simulink model "uncontrolledRectifier"  (R2021a)
settings: Solver=ode23t  StartTime=0.0  StopTime=.1  FixedStep=.000001  MaxStep=.0001  RelTol=1e-3
undefined symbols (not defined in the file): D1, D11, Delta
libraries: spsVoltageMeasurementLib x49, spsDiodeLib x45, spsCurrentMeasurementLib x21, spsACVoltageSourceLib x20, spsSeriesRLCBranchLib x17, spsMeanLib x3, spsGroundLib x2, spsPowerLib x2, spsThreePhaseTransformerThreeWindingsLib x1, spspowerguiLib x1
settings Model: Creator=User  LastModifiedBy=User

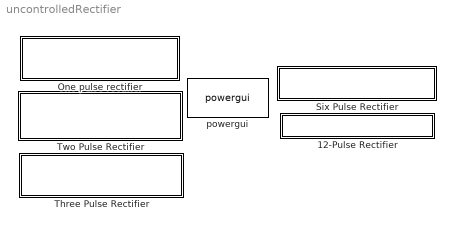
== system uncontrolledRectifier ==
  12-Pulse Rectifier : Subsystem
  One pulse rectifier : Subsystem
  Six Pulse Rectifier : Subsystem
  Three Pulse Rectifier : Subsystem
  Two Pulse Rectifier : Subsystem
  powergui : spspowerguiLib/powergui  Priority=1  SimulationMode=Continuous  SampleTime=50e-6  frequency=60  Iterations=50  frequencyindice=50  Pbase=100e6  ErrMax=1e-4  UnitsV=kV  UnitsW=MW  buscounter=0  FunctionMessages=off  echomessages=off  EnableUseOfTLC=off  CurrentSourceSwitches=off  DisableSnubberDevices=off  DisableRonSwitches=off  DisableVfSwitches=off  DisplayEquations=off  AutomaticDiscreteSolvers=off  SolverType=Tustin/Backward Euler (TBE)  Interpol=off  ExternalGateDelay=off  methode=off  Ts=100  x0status=blocks  SPID=on  SwTol=0  HookPort=off  NonlinearTolerance=1e-4  nMaxIteration=100  ContinueOnMaxIteration=off  RestoreLinks=warning  ResistiveCurrentMeasurement=off  Frange=[0:2:500]  Ylog=off  Xlog=on  ShowGrid=off  save=off  variable=ZData  structure=0  ZoomFFT=off  StartTime=0.0  cycles=1  DisplayStyle=1  fundamental=60  FreqAxis=off  MaxFrequency=1000  frequencyindicesteady=1  RmsSteady=1  display=off

== system uncontrolledRectifier/12-Pulse Rectifier ==
  Subsystem : Subsystem

== system uncontrolledRectifier/One pulse rectifier ==
  Half Wave RL & FWD : Subsystem
  Half Wave RL load : Subsystem
  Half Wave with R : Subsystem
  Half Wave with R//C : Subsystem

== system uncontrolledRectifier/Six Pulse Rectifier ==
  6-pulse with R load : Subsystem
  6-pulse with RL load : Subsystem

== system uncontrolledRectifier/Three Pulse Rectifier ==
  R load : Subsystem

== system uncontrolledRectifier/Two Pulse Rectifier ==
  Full wave with R load : Subsystem
  Full wave with R load And C filter : Subsystem
  Full wave with RL load : Subsystem

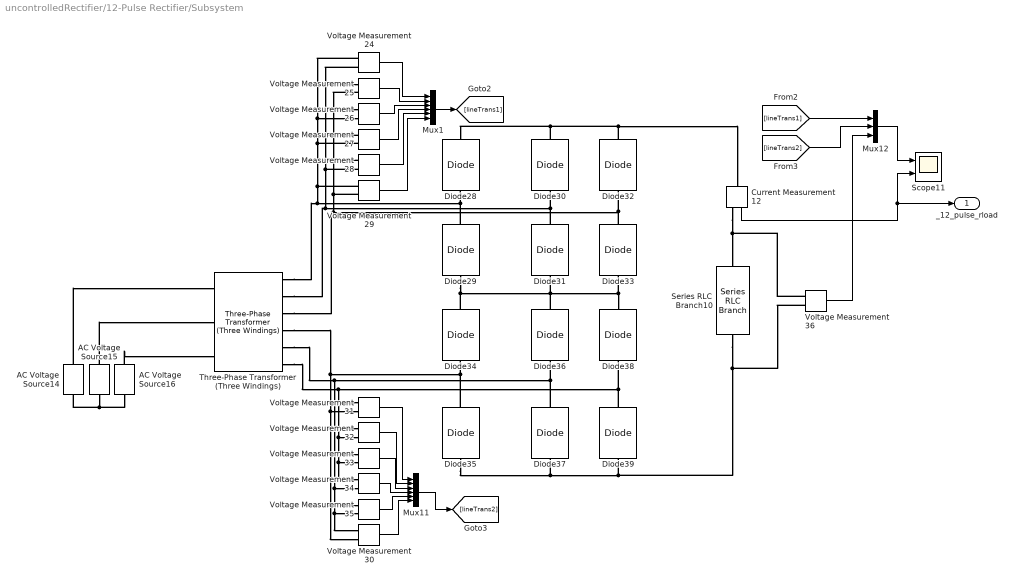
== system uncontrolledRectifier/12-Pulse Rectifier/Subsystem ==
  AC Voltage Source14 : spsACVoltageSourceLib/AC Voltage Source  Amplitude=220*sqrt(2)  Phase=0  Frequency=50  SampleTime=0  Measurements=None  BusType=swing  Pref=10e3  Qref=0  Qmin=-inf  Qmax=+inf
  AC Voltage Source15 : spsACVoltageSourceLib/AC Voltage Source  Amplitude=220*sqrt(2)  Phase=-120  Frequency=50  SampleTime=0  Measurements=None  BusType=swing  Pref=10e3  Qref=0  Qmin=-inf  Qmax=+inf
  AC Voltage Source16 : spsACVoltageSourceLib/AC Voltage Source  Amplitude=220*sqrt(2)  Phase=120  Frequency=50  SampleTime=0  Measurements=None  BusType=swing  Pref=10e3  Qref=0  Qmin=-inf  Qmax=+inf
  Current Measurement12 : spsCurrentMeasurementLib/Current Measurement  PhasorSimulation=off  OutputType=Complex  PSBequivalent=0
  Diode{28..39} (12 alike) : spsDiodeLib/Diode  Ron=0.001  Lon=0  Vf=0.8  IC=0  UseSnubber=0  Rs=500  Cs=250e-9  Measurements=off
  Mux1 : Mux  Inputs=6
  Mux11 : Mux  Inputs=6
  Mux12 : Mux  Inputs=3
  Scope11 : Scope  NumInputPorts=2
  Series RLC Branch10 : spsSeriesRLCBranchLib/Series RLC Branch  LConnTagsString=__new0  RConnTagsString=__new0  BranchType=R  Resistance=10  Inductance=1e-3  SetiL0=off  InitialCurrent=0  Capacitance=1e-6  Setx0=off  InitialVoltage=0  Measurements=None
  Three-Phase Transformer (Three Windings) : spsThreePhaseTransformerThreeWindingsLib/Three-Phase Transformer (Three Windings)  Winding1Connection=Delta (D1)  Winding2Connection=Y  Winding3Connection=Delta (D11)  CoreType=Three single-phase transformers  SetSaturation=off  Hysteresis=off  DataFile='hysteresis'  SetInitialFlux=off  Measurements=None  UNITS=pu  NominalPower=[ 6000 , 50 ]  Winding1=[ 380 , 0.002 , 0.08 ]  Winding2=[ 100 , 0.002 , 0.08 ]  Winding3=[ 100 , 0.002 , 0.08 ]  Rm=500  Lm=500  L0=0.5  Saturation=[ 0,0 ; 0.0024,1.2 ; 1.0,1.52 ]  InitialFluxes=[0.8 -0.8 0.7]  BreakLoop=off  DiscreteSolver=Trapezoidal iterative  DataType=off  TransfoNumber=1
      settings: SourceProductBaseCode=PS
  Voltage Measurement{24..36} (13 alike) : spsVoltageMeasurementLib/Voltage Measurement  PhasorSimulation=off  OutputType=Complex  PSBequivalent=0
  _12_pulse_rload : Outport
  wires:
  Voltage Measurement36/1 -> Mux12/3
  Mux12/1 -> Scope11/1
  Voltage Measurement33/1 -> Mux11/3
  Voltage Measurement24/1 -> Mux1/1
  Voltage Measurement25/1 -> Mux1/2
  Voltage Measurement29/1 -> Mux1/6
  Mux1/1 -> [lineTrans1]
  Voltage Measurement26/1 -> Mux1/3
  Voltage Measurement34/1 -> Mux11/4
  Voltage Measurement30/1 -> Mux11/6
  Voltage Measurement31/1 -> Mux11/1
  Voltage Measurement28/1 -> Mux1/5
  Voltage Measurement35/1 -> Mux11/5
  [lineTrans1] -> Mux12/1
  Mux11/1 -> [lineTrans2]
  Current Measurement12/1 -> _12_pulse_rload/1, Scope11/2
  [lineTrans2] -> Mux12/2
  Voltage Measurement32/1 -> Mux11/2
  Voltage Measurement27/1 -> Mux1/4
  connections:
  Diode37/RConn1 -- Three-Phase Transformer (Three Windings)/RConn5 -- Voltage Measurement33/LConn1 -- Voltage Measurement35/LConn2 -- Voltage Measurement30/LConn1 -- Voltage Measurement34/LConn2 -- Diode36/LConn1
  Diode35/RConn1 -- Voltage Measurement32/LConn1 -- Voltage Measurement35/LConn1 -- Voltage Measurement30/LConn2 -- Voltage Measurement31/LConn2 -- Three-Phase Transformer (Three Windings)/RConn4 -- Diode34/LConn1
  AC Voltage Source15/LConn1 -- AC Voltage Source16/LConn1 -- AC Voltage Source14/LConn1
  Diode33/RConn1 -- Voltage Measurement29/LConn2 -- Voltage Measurement25/LConn2 -- Voltage Measurement26/LConn1 -- Three-Phase Transformer (Three Windings)/RConn3 -- Diode32/LConn1
  AC Voltage Source16/RConn1 -- Three-Phase Transformer (Three Windings)/LConn3
  Diode36/RConn1 -- Diode34/RConn1 -- Diode29/LConn1 -- Diode31/LConn1 -- Diode33/LConn1 -- Diode38/RConn1
  Diode30/RConn1 -- Current Measurement12/LConn1 -- Diode32/RConn1 -- Diode28/RConn1
  Diode39/RConn1 -- Voltage Measurement31/LConn1 -- Voltage Measurement32/LConn2 -- Voltage Measurement33/LConn2 -- Voltage Measurement34/LConn1 -- Three-Phase Transformer (Three Windings)/RConn6 -- Diode38/LConn1
  Diode31/RConn1 -- Voltage Measurement28/LConn2 -- Voltage Measurement27/LConn1 -- Voltage Measurement24/LConn2 -- Voltage Measurement25/LConn1 -- Three-Phase Transformer (Three Windings)/RConn2 -- Diode30/LConn1
  AC Voltage Source14/RConn1 -- Three-Phase Transformer (Three Windings)/LConn1
  Current Measurement12/RConn1 -- Voltage Measurement36/LConn1 -- Series RLC Branch10/LConn1
  Diode35/LConn1 -- Diode37/LConn1 -- Voltage Measurement36/LConn2 -- Series RLC Branch10/RConn1 -- Diode39/LConn1
  Diode29/RConn1 -- Voltage Measurement29/LConn1 -- Voltage Measurement28/LConn1 -- Voltage Measurement27/LConn2 -- Voltage Measurement26/LConn2 -- Voltage Measurement24/LConn1 -- Three-Phase Transformer (Three Windings)/RConn1 -- Diode28/LConn1
  AC Voltage Source15/RConn1 -- Three-Phase Transformer (Three Windings)/LConn2

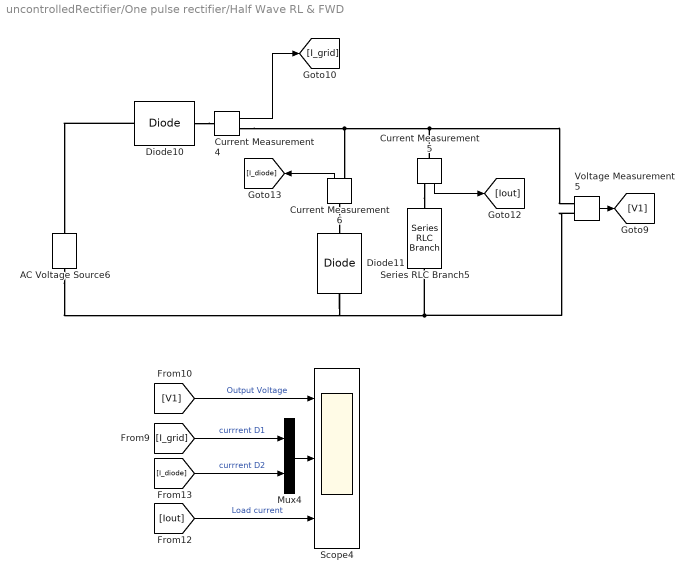
== system uncontrolledRectifier/One pulse rectifier/Half Wave RL & FWD ==
  AC Voltage Source6 : spsACVoltageSourceLib/AC Voltage Source  Amplitude=220  Phase=0  Frequency=50  SampleTime=0  Measurements=None  BusType=swing  Pref=10e3  Qref=0  Qmin=-inf  Qmax=+inf
  Current Measurement4 : spsCurrentMeasurementLib/Current Measurement  PhasorSimulation=off  OutputType=Complex  PSBequivalent=0
  Current Measurement5 : spsCurrentMeasurementLib/Current Measurement  PhasorSimulation=off  OutputType=Complex  PSBequivalent=0
  Current Measurement6 : spsCurrentMeasurementLib/Current Measurement  PhasorSimulation=off  OutputType=Complex  PSBequivalent=0
  Diode10 : spsDiodeLib/Diode  Ron=0.001  Lon=0  Vf=0.8  IC=0  UseSnubber=0  Rs=500  Cs=250e-9  Measurements=off
  Diode11 : spsDiodeLib/Diode  Ron=0.001  Lon=0  Vf=0.8  IC=0  UseSnubber=0  Rs=500  Cs=250e-9  Measurements=off
  Mux4 : Mux  Inputs=2
  Scope4 : Scope  NumInputPorts=3
  Series RLC Branch5 : spsSeriesRLCBranchLib/Series RLC Branch  LConnTagsString=__new0  RConnTagsString=__new0  BranchType=RL  Resistance=10  Inductance=1  SetiL0=off  InitialCurrent=0  Capacitance=1e-6  Setx0=off  InitialVoltage=0  Measurements=None
  Voltage Measurement5 : spsVoltageMeasurementLib/Voltage Measurement  PhasorSimulation=off  OutputType=Complex  PSBequivalent=0
  wires:
  [V1] -> Scope4/1  "Output Voltage"
  Mux4/1 -> Scope4/2
  Current Measurement6/1 -> [I_diode]
  Current Measurement5/1 -> [Iout]
  Current Measurement4/1 -> [I_grid]
  [I_grid] -> Mux4/1  "currrent D1"
  Voltage Measurement5/1 -> [V1]
  [Iout] -> Scope4/3  "Load current"
  [I_diode] -> Mux4/2  "currrent D2"
  connections:
  Voltage Measurement5/LConn2 -- Diode11/LConn1 -- AC Voltage Source6/LConn1 -- Series RLC Branch5/RConn1
  Diode10/LConn1 -- AC Voltage Source6/RConn1
  Current Measurement4/RConn1 -- Current Measurement5/LConn1 -- Voltage Measurement5/LConn1 -- Current Measurement6/RConn1
  Current Measurement5/RConn1 -- Series RLC Branch5/LConn1
  Diode10/RConn1 -- Current Measurement4/LConn1
  Current Measurement6/LConn1 -- Diode11/RConn1

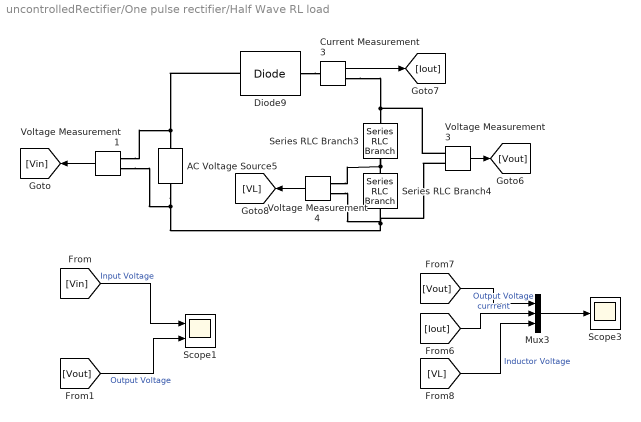
== system uncontrolledRectifier/One pulse rectifier/Half Wave RL load ==
  AC Voltage Source5 : spsACVoltageSourceLib/AC Voltage Source  Amplitude=220  Phase=0  Frequency=50  SampleTime=0  Measurements=None  BusType=swing  Pref=10e3  Qref=0  Qmin=-inf  Qmax=+inf
  Current Measurement3 : spsCurrentMeasurementLib/Current Measurement  PhasorSimulation=off  OutputType=Complex  PSBequivalent=0
  Diode9 : spsDiodeLib/Diode  Ron=0.001  Lon=0  Vf=0.8  IC=0  UseSnubber=0  Rs=500  Cs=250e-9  Measurements=off
  Mux3 : Mux  Inputs=3
  Scope1 : Scope  NumInputPorts=2
  Scope3 : Scope
  Series RLC Branch3 : spsSeriesRLCBranchLib/Series RLC Branch  LConnTagsString=__new0  RConnTagsString=__new0  BranchType=R  Resistance=10  Inductance=1e-3  SetiL0=off  InitialCurrent=0  Capacitance=1e-6  Setx0=off  InitialVoltage=0  Measurements=None
  Series RLC Branch4 : spsSeriesRLCBranchLib/Series RLC Branch  LConnTagsString=__new0  RConnTagsString=__new0  BranchType=L  Resistance=10  Inductance=10/(2*pi*50)  SetiL0=off  InitialCurrent=0  Capacitance=1e-6  Setx0=off  InitialVoltage=0  Measurements=None
  Voltage Measurement1 : spsVoltageMeasurementLib/Voltage Measurement  PhasorSimulation=off  OutputType=Complex  PSBequivalent=0
  Voltage Measurement3 : spsVoltageMeasurementLib/Voltage Measurement  PhasorSimulation=off  OutputType=Complex  PSBequivalent=0
  Voltage Measurement4 : spsVoltageMeasurementLib/Voltage Measurement  PhasorSimulation=off  OutputType=Complex  PSBequivalent=0
  wires:
  [Vout] -> Mux3/1  "Output Voltage"
  Current Measurement3/1 -> [Iout]
  Voltage Measurement3/1 -> [Vout]
  [Iout] -> Mux3/2  "currrent"
  Voltage Measurement4/1 -> [VL]
  [VL] -> Mux3/3  "Inductor Voltage"
  Mux3/1 -> Scope3/1
  Voltage Measurement1/1 -> [Vin]
  [Vin] -> Scope1/1  "Input Voltage"
  [Vout] -> Scope1/2  "Output Voltage"
  connections:
  AC Voltage Source5/LConn1 -- Voltage Measurement1/LConn2 -- Voltage Measurement4/LConn2 -- Voltage Measurement3/LConn2 -- Series RLC Branch4/RConn1
  Series RLC Branch4/LConn1 -- Voltage Measurement4/LConn1 -- Series RLC Branch3/RConn1
  Current Measurement3/RConn1 -- Voltage Measurement3/LConn1 -- Series RLC Branch3/LConn1
  Diode9/RConn1 -- Current Measurement3/LConn1
  Diode9/LConn1 -- Voltage Measurement1/LConn1 -- AC Voltage Source5/RConn1

== system uncontrolledRectifier/One pulse rectifier/Half Wave with R ==
  AC Voltage Source : spsACVoltageSourceLib/AC Voltage Source  Amplitude=220  Phase=0  Frequency=50  SampleTime=0  Measurements=None  BusType=swing  Pref=10e3  Qref=0  Qmin=-inf  Qmax=+inf
  Current Measurement : spsCurrentMeasurementLib/Current Measurement  PhasorSimulation=off  OutputType=Complex  PSBequivalent=0
  Diode1 : spsDiodeLib/Diode  Ron=0.001  Lon=0  Vf=0.8  IC=0  UseSnubber=0  Rs=500  Cs=250e-9  Measurements=off
  Scope : Scope  NumInputPorts=2
  Scope1 : Scope
  Series RLC Branch : spsSeriesRLCBranchLib/Series RLC Branch  LConnTagsString=__new0  RConnTagsString=__new0  BranchType=R  Resistance=10  Inductance=1e-3  SetiL0=off  InitialCurrent=0  Capacitance=1e-6  Setx0=off  InitialVoltage=0  Measurements=None
  Voltage Measurement : spsVoltageMeasurementLib/Voltage Measurement  PhasorSimulation=off  OutputType=Complex  PSBequivalent=0
  Voltage Measurement1 : spsVoltageMeasurementLib/Voltage Measurement  PhasorSimulation=off  OutputType=Complex  PSBequivalent=0
  wires:
  Current Measurement/1 -> Scope/1  "Iout"
  Voltage Measurement/1 -> Scope/2  "Vout"
  Voltage Measurement1/1 -> Scope1/1  "Vd"
  connections:
  AC Voltage Source/LConn1 -- Voltage Measurement/LConn2 -- Series RLC Branch/RConn1
  Diode1/LConn1 -- Voltage Measurement1/LConn1 -- AC Voltage Source/RConn1
  Voltage Measurement/LConn1 -- Current Measurement/RConn1 -- Series RLC Branch/LConn1
  Diode1/RConn1 -- Voltage Measurement1/LConn2 -- Current Measurement/LConn1

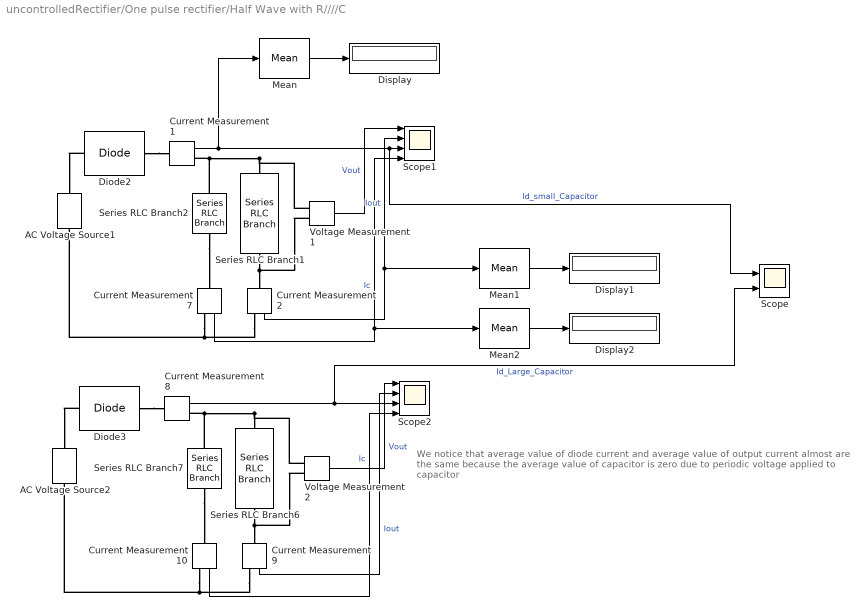
== system uncontrolledRectifier/One pulse rectifier/Half Wave with R////C ==
  note: We notice that average value of diode current and average value of output current almost are the same because the average value of capacitor is zero due to periodic voltage applied to capacitor
  AC Voltage Source1 : spsACVoltageSourceLib/AC Voltage Source  Amplitude=220  Phase=0  Frequency=50  SampleTime=0  Measurements=None  BusType=swing  Pref=10e3  Qref=0  Qmin=-inf  Qmax=+inf
  AC Voltage Source2 : spsACVoltageSourceLib/AC Voltage Source  Amplitude=220  Phase=0  Frequency=50  SampleTime=0  Measurements=None  BusType=swing  Pref=10e3  Qref=0  Qmin=-inf  Qmax=+inf
  Current Measurement{1..2,7..10} (6 alike) : spsCurrentMeasurementLib/Current Measurement  PhasorSimulation=off  OutputType=Complex  PSBequivalent=0
  Diode2 : spsDiodeLib/Diode  Ron=0.001  Lon=0  Vf=0.8  IC=0  UseSnubber=0  Rs=500  Cs=250e-9  Measurements=off
  Diode3 : spsDiodeLib/Diode  Ron=0.001  Lon=0  Vf=0.8  IC=0  UseSnubber=0  Rs=500  Cs=250e-9  Measurements=off
  Display : Display
  Display1 : Display
  Display2 : Display
  Mean : spsMeanLib/Mean  Freq=60  Vinit=0  Ts=0
  Mean1 : spsMeanLib/Mean  Freq=60  Vinit=0  Ts=0
  Mean2 : spsMeanLib/Mean  Freq=60  Vinit=0  Ts=0
  Scope : Scope  NumInputPorts=2
  Scope1 : Scope  NumInputPorts=4
  Scope2 : Scope  NumInputPorts=4
  Series RLC Branch1 : spsSeriesRLCBranchLib/Series RLC Branch  LConnTagsString=__new0  RConnTagsString=__new0  BranchType=R  Resistance=10  Inductance=1e-3  SetiL0=off  InitialCurrent=0  Capacitance=1e-6  Setx0=off  InitialVoltage=0  Measurements=None
  Series RLC Branch2 : spsSeriesRLCBranchLib/Series RLC Branch  LConnTagsString=__new0  RConnTagsString=__new0  BranchType=C  Resistance=10  Inductance=1e-3  SetiL0=off  InitialCurrent=0  Capacitance=10e-3  Setx0=off  InitialVoltage=0  Measurements=None
  Series RLC Branch6 : spsSeriesRLCBranchLib/Series RLC Branch  LConnTagsString=__new0  RConnTagsString=__new0  BranchType=R  Resistance=10  Inductance=1e-3  SetiL0=off  InitialCurrent=0  Capacitance=1e-6  Setx0=off  InitialVoltage=0  Measurements=None
  Series RLC Branch7 : spsSeriesRLCBranchLib/Series RLC Branch  LConnTagsString=__new0  RConnTagsString=__new0  BranchType=C  Resistance=10  Inductance=1e-3  SetiL0=off  InitialCurrent=0  Capacitance=50e-3  Setx0=off  InitialVoltage=0  Measurements=None
  Voltage Measurement1 : spsVoltageMeasurementLib/Voltage Measurement  PhasorSimulation=off  OutputType=Complex  PSBequivalent=0
  Voltage Measurement2 : spsVoltageMeasurementLib/Voltage Measurement  PhasorSimulation=off  OutputType=Complex  PSBequivalent=0
  wires:
  Voltage Measurement2/1 -> Scope2/1  "Vout"
  Current Measurement7/1 -> Mean2/1, Scope1/4  "Ic"
  Voltage Measurement1/1 -> Scope1/1  "Vout"
  Current Measurement8/1 -> Scope/2, Scope2/3  "Id_Large_Capacitor"
  Mean/1 -> Display/1
  Current Measurement10/1 -> Scope2/4  "Ic"
  Mean1/1 -> Display1/1
  Mean2/1 -> Display2/1
  Current Measurement1/1 -> Mean/1, Scope/1, Scope1/3  "Id_small_Capacitor"
  Current Measurement9/1 -> Scope2/2  "Iout"
  Current Measurement2/1 -> Mean1/1, Scope1/2  "Iout"
  connections:
  Diode2/LConn1 -- AC Voltage Source1/RConn1
  Series RLC Branch2/RConn1 -- Current Measurement7/LConn1
  Diode3/RConn1 -- Current Measurement8/LConn1
  Current Measurement2/RConn1 -- Current Measurement7/RConn1 -- AC Voltage Source1/LConn1
  Current Measurement1/RConn1 -- Voltage Measurement1/LConn1 -- Series RLC Branch1/LConn1 -- Series RLC Branch2/LConn1
  Current Measurement9/RConn1 -- Current Measurement10/RConn1 -- AC Voltage Source2/LConn1
  Diode2/RConn1 -- Current Measurement1/LConn1
  Voltage Measurement1/LConn2 -- Current Measurement2/LConn1 -- Series RLC Branch1/RConn1
  Voltage Measurement2/LConn2 -- Series RLC Branch6/RConn1 -- Current Measurement9/LConn1
  Diode3/LConn1 -- AC Voltage Source2/RConn1
  Series RLC Branch7/LConn1 -- Current Measurement8/RConn1 -- Voltage Measurement2/LConn1 -- Series RLC Branch6/LConn1
  Series RLC Branch7/RConn1 -- Current Measurement10/LConn1

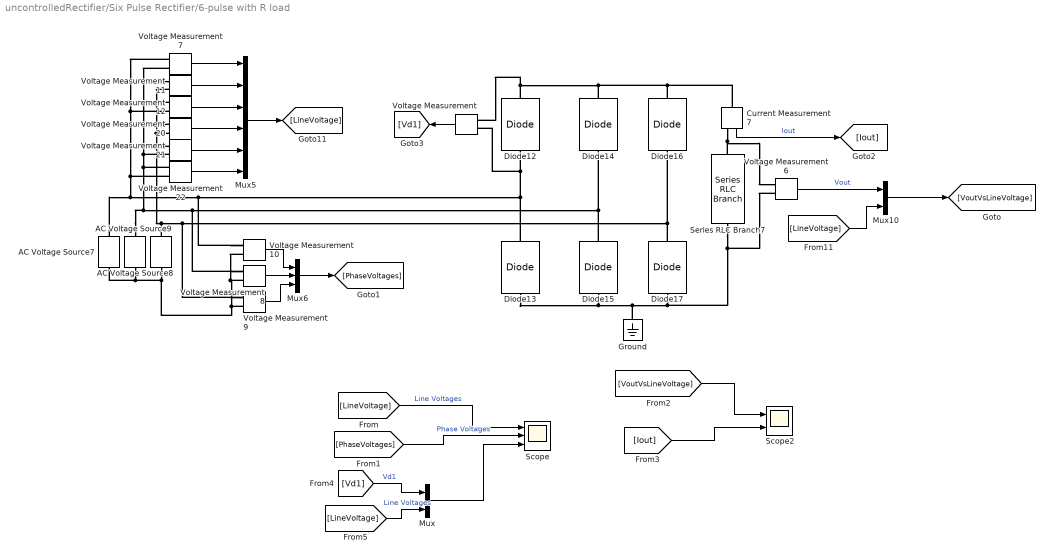
== system uncontrolledRectifier/Six Pulse Rectifier/6-pulse with R load ==
  AC Voltage Source7 : spsACVoltageSourceLib/AC Voltage Source  Amplitude=220  Phase=0  Frequency=50  SampleTime=0  Measurements=None  BusType=swing  Pref=10e3  Qref=0  Qmin=-inf  Qmax=+inf
  AC Voltage Source8 : spsACVoltageSourceLib/AC Voltage Source  Amplitude=220  Phase=-120  Frequency=50  SampleTime=0  Measurements=None  BusType=swing  Pref=10e3  Qref=0  Qmin=-inf  Qmax=+inf
  AC Voltage Source9 : spsACVoltageSourceLib/AC Voltage Source  Amplitude=220  Phase=120  Frequency=50  SampleTime=0  Measurements=None  BusType=swing  Pref=10e3  Qref=0  Qmin=-inf  Qmax=+inf
  Current Measurement7 : spsCurrentMeasurementLib/Current Measurement  PhasorSimulation=off  OutputType=Complex  PSBequivalent=0
  Diode{12..17} (6 alike) : spsDiodeLib/Diode  Ron=0.001  Lon=0  Vf=0.8  IC=0  UseSnubber=0  Rs=500  Cs=250e-9  Measurements=off
  Ground : spsGroundLib/Ground  LConnTagsString=a
  Mux : Mux  Inputs=2
  Mux10 : Mux  Inputs=2
  Mux5 : Mux  Inputs=6
  Mux6 : Mux  Inputs=3
  Scope : Scope  NumInputPorts=3
  Scope2 : Scope  NumInputPorts=2
  Series RLC Branch7 : spsSeriesRLCBranchLib/Series RLC Branch  LConnTagsString=__new0  RConnTagsString=__new0  BranchType=R  Resistance=10  Inductance=1e-3  SetiL0=off  InitialCurrent=0  Capacitance=1e-6  Setx0=off  InitialVoltage=0  Measurements=None
  Voltage Measurement{,6..12,20..22} (11 alike) : spsVoltageMeasurementLib/Voltage Measurement  PhasorSimulation=off  OutputType=Complex  PSBequivalent=0
  wires:
  Mux10/1 -> [VoutVsLineVoltage]
  Current Measurement7/1 -> [Iout]  "Iout"
  Mux5/1 -> [LineVoltage]
  Voltage Measurement7/1 -> Mux5/1
  Voltage Measurement9/1 -> Mux6/3
  Voltage Measurement21/1 -> Mux5/5
  Voltage Measurement11/1 -> Mux5/2
  Voltage Measurement22/1 -> Mux5/6
  Voltage Measurement6/1 -> Mux10/1  "Vout"
  Voltage Measurement10/1 -> Mux6/1
  Voltage Measurement8/1 -> Mux6/2
  [LineVoltage] -> Mux10/2
  Voltage Measurement12/1 -> Mux5/3
  Voltage Measurement20/1 -> Mux5/4
  Mux6/1 -> [PhaseVoltages]
  [LineVoltage] -> Scope/1  "Line Voltages"
  [PhaseVoltages] -> Scope/2  "Phase Voltages"
  [VoutVsLineVoltage] -> Scope2/1
  [Iout] -> Scope2/2
  Voltage Measurement/1 -> [Vd1]
  [Vd1] -> Mux/1  "Vd1"
  [LineVoltage] -> Mux/2  "Line Voltages"
  Mux/1 -> Scope/3
  connections:
  AC Voltage Source8/RConn1 -- Voltage Measurement22/LConn1 -- Voltage Measurement7/LConn2 -- Voltage Measurement11/LConn1 -- Voltage Measurement21/LConn2 -- Voltage Measurement8/LConn1 -- Diode15/RConn1 -- Diode14/LConn1
  Current Measurement7/LConn1 -- Diode16/RConn1 -- Voltage Measurement/LConn2 -- Diode12/RConn1 -- Diode14/RConn1
  AC Voltage Source9/RConn1 -- Voltage Measurement20/LConn2 -- Voltage Measurement12/LConn1 -- Voltage Measurement11/LConn2 -- Voltage Measurement21/LConn1 -- Voltage Measurement9/LConn1 -- Diode17/RConn1 -- Diode16/LConn1
  Series RLC Branch7/LConn1 -- Current Measurement7/RConn1 -- Voltage Measurement6/LConn1
  Diode15/LConn1 -- Diode13/LConn1 -- Ground/LConn1 -- Voltage Measurement6/LConn2 -- Series RLC Branch7/RConn1 -- Diode17/LConn1
  AC Voltage Source8/LConn1 -- AC Voltage Source9/LConn1 -- Voltage Measurement10/LConn2 -- Voltage Measurement8/LConn2 -- Voltage Measurement9/LConn2 -- AC Voltage Source7/LConn1
  AC Voltage Source7/RConn1 -- Voltage Measurement22/LConn2 -- Voltage Measurement12/LConn2 -- Voltage Measurement7/LConn1 -- Voltage Measurement20/LConn1 -- Voltage Measurement10/LConn1 -- Diode12/LConn1 -- Voltage Measurement/LConn1 -- Diode13/RConn1

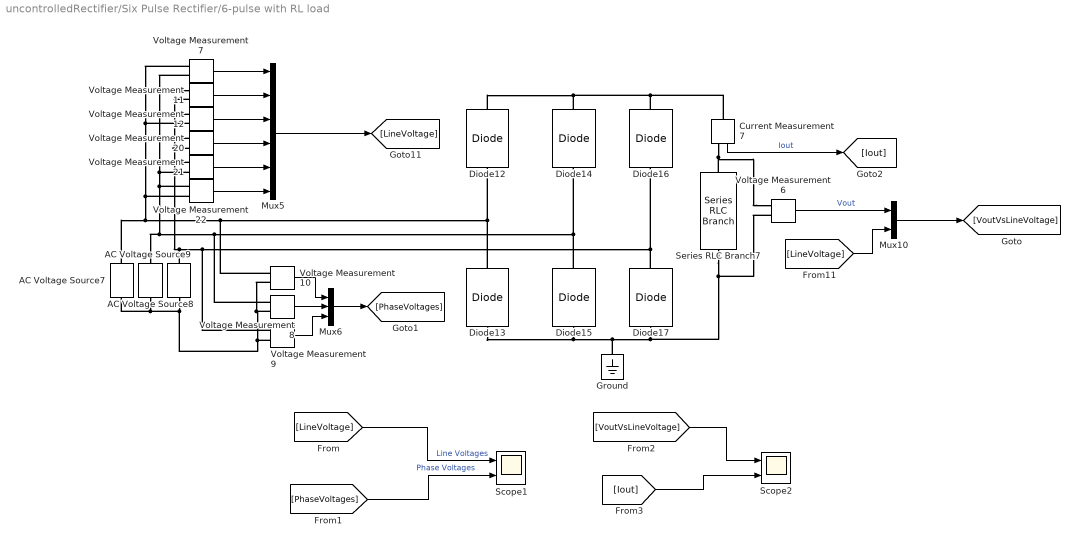
== system uncontrolledRectifier/Six Pulse Rectifier/6-pulse with RL load ==
  AC Voltage Source7 : spsACVoltageSourceLib/AC Voltage Source  Amplitude=220  Phase=0  Frequency=50  SampleTime=0  Measurements=None  BusType=swing  Pref=10e3  Qref=0  Qmin=-inf  Qmax=+inf
  AC Voltage Source8 : spsACVoltageSourceLib/AC Voltage Source  Amplitude=220  Phase=-120  Frequency=50  SampleTime=0  Measurements=None  BusType=swing  Pref=10e3  Qref=0  Qmin=-inf  Qmax=+inf
  AC Voltage Source9 : spsACVoltageSourceLib/AC Voltage Source  Amplitude=220  Phase=120  Frequency=50  SampleTime=0  Measurements=None  BusType=swing  Pref=10e3  Qref=0  Qmin=-inf  Qmax=+inf
  Current Measurement7 : spsCurrentMeasurementLib/Current Measurement  PhasorSimulation=off  OutputType=Complex  PSBequivalent=0
  Diode{12..17} (6 alike) : spsDiodeLib/Diode  Ron=0.001  Lon=0  Vf=0.8  IC=0  UseSnubber=0  Rs=500  Cs=250e-9  Measurements=off
  Ground : spsGroundLib/Ground  LConnTagsString=a
  Mux10 : Mux  Inputs=2
  Mux5 : Mux  Inputs=6
  Mux6 : Mux  Inputs=3
  Scope1 : Scope  NumInputPorts=2
  Scope2 : Scope  NumInputPorts=2
  Series RLC Branch7 : spsSeriesRLCBranchLib/Series RLC Branch  LConnTagsString=__new0  RConnTagsString=__new0  BranchType=RL  Resistance=10  Inductance=100e-3  SetiL0=off  InitialCurrent=0  Capacitance=1e-6  Setx0=off  InitialVoltage=0  Measurements=None
  Voltage Measurement{6..12,20..22} (10 alike) : spsVoltageMeasurementLib/Voltage Measurement  PhasorSimulation=off  OutputType=Complex  PSBequivalent=0
  wires:
  [LineVoltage] -> Scope1/1  "Line Voltages"
  Mux6/1 -> [PhaseVoltages]
  Current Measurement7/1 -> [Iout]  "Iout"
  [LineVoltage] -> Mux10/2
  Voltage Measurement20/1 -> Mux5/4
  Voltage Measurement8/1 -> Mux6/2
  Voltage Measurement10/1 -> Mux6/1
  Voltage Measurement6/1 -> Mux10/1  "Vout"
  Voltage Measurement12/1 -> Mux5/3
  Voltage Measurement22/1 -> Mux5/6
  Mux10/1 -> [VoutVsLineVoltage]
  Mux5/1 -> [LineVoltage]
  [Iout] -> Scope2/2
  [VoutVsLineVoltage] -> Scope2/1
  Voltage Measurement9/1 -> Mux6/3
  Voltage Measurement7/1 -> Mux5/1
  Voltage Measurement21/1 -> Mux5/5
  [PhaseVoltages] -> Scope1/2  "Phase Voltages"
  Voltage Measurement11/1 -> Mux5/2
  connections:
  Diode16/LConn1 -- Diode17/RConn1 -- Voltage Measurement9/LConn1 -- AC Voltage Source9/RConn1 -- Voltage Measurement20/LConn2 -- Voltage Measurement12/LConn1 -- Voltage Measurement11/LConn2 -- Voltage Measurement21/LConn1
  Diode12/RConn1 -- Diode14/RConn1 -- Current Measurement7/LConn1 -- Diode16/RConn1
  Diode14/LConn1 -- Diode15/RConn1 -- Voltage Measurement8/LConn1 -- AC Voltage Source8/RConn1 -- Voltage Measurement22/LConn1 -- Voltage Measurement7/LConn2 -- Voltage Measurement11/LConn1 -- Voltage Measurement21/LConn2
  AC Voltage Source7/LConn1 -- AC Voltage Source8/LConn1 -- AC Voltage Source9/LConn1 -- Voltage Measurement10/LConn2 -- Voltage Measurement8/LConn2 -- Voltage Measurement9/LConn2
  Diode13/RConn1 -- Diode12/LConn1 -- Voltage Measurement10/LConn1 -- AC Voltage Source7/RConn1 -- Voltage Measurement22/LConn2 -- Voltage Measurement12/LConn2 -- Voltage Measurement7/LConn1 -- Voltage Measurement20/LConn1
  Voltage Measurement6/LConn1 -- Series RLC Branch7/LConn1 -- Current Measurement7/RConn1
  Diode17/LConn1 -- Diode15/LConn1 -- Diode13/LConn1 -- Ground/LConn1 -- Voltage Measurement6/LConn2 -- Series RLC Branch7/RConn1

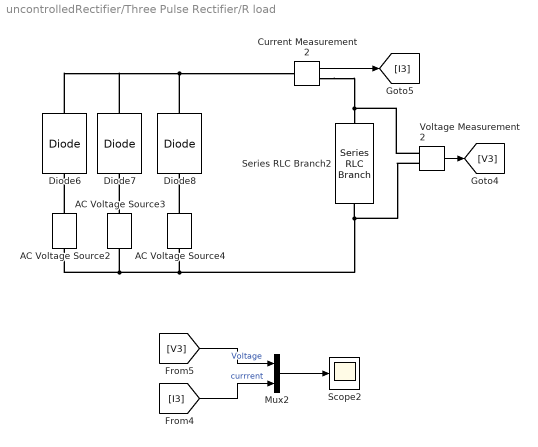
== system uncontrolledRectifier/Three Pulse Rectifier/R load ==
  AC Voltage Source2 : spsACVoltageSourceLib/AC Voltage Source  Amplitude=220  Phase=0  Frequency=50  SampleTime=0  Measurements=None  BusType=swing  Pref=10e3  Qref=0  Qmin=-inf  Qmax=+inf
  AC Voltage Source3 : spsACVoltageSourceLib/AC Voltage Source  Amplitude=220  Phase=120  Frequency=50  SampleTime=0  Measurements=None  BusType=swing  Pref=10e3  Qref=0  Qmin=-inf  Qmax=+inf
  AC Voltage Source4 : spsACVoltageSourceLib/AC Voltage Source  Amplitude=220  Phase=240  Frequency=50  SampleTime=0  Measurements=None  BusType=swing  Pref=10e3  Qref=0  Qmin=-inf  Qmax=+inf
  Current Measurement2 : spsCurrentMeasurementLib/Current Measurement  PhasorSimulation=off  OutputType=Complex  PSBequivalent=0
  Diode6 : spsDiodeLib/Diode  Ron=0.001  Lon=0  Vf=0.8  IC=0  UseSnubber=0  Rs=500  Cs=250e-9  Measurements=off
  Diode7 : spsDiodeLib/Diode  Ron=0.001  Lon=0  Vf=0.8  IC=0  UseSnubber=0  Rs=500  Cs=250e-9  Measurements=off
  Diode8 : spsDiodeLib/Diode  Ron=0.001  Lon=0  Vf=0.8  IC=0  UseSnubber=0  Rs=500  Cs=250e-9  Measurements=off
  Mux2 : Mux  Inputs=2
  Scope2 : Scope
  Series RLC Branch2 : spsSeriesRLCBranchLib/Series RLC Branch  LConnTagsString=__new0  RConnTagsString=__new0  BranchType=R  Resistance=10  Inductance=1e-3  SetiL0=off  InitialCurrent=0  Capacitance=1e-6  Setx0=off  InitialVoltage=0  Measurements=None
  Voltage Measurement2 : spsVoltageMeasurementLib/Voltage Measurement  PhasorSimulation=off  OutputType=Complex  PSBequivalent=0
  wires:
  Current Measurement2/1 -> [I3]
  [I3] -> Mux2/2  "currrent"
  [V3] -> Mux2/1  "Voltage"
  Mux2/1 -> Scope2/1
  Voltage Measurement2/1 -> [V3]
  connections:
  Voltage Measurement2/LConn2 -- AC Voltage Source2/LConn1 -- AC Voltage Source3/LConn1 -- AC Voltage Source4/LConn1 -- Series RLC Branch2/RConn1
  AC Voltage Source4/RConn1 -- Diode8/LConn1
  AC Voltage Source2/RConn1 -- Diode6/LConn1
  AC Voltage Source3/RConn1 -- Diode7/LConn1
  Diode8/RConn1 -- Diode7/RConn1 -- Diode6/RConn1 -- Current Measurement2/LConn1
  Voltage Measurement2/LConn1 -- Current Measurement2/RConn1 -- Series RLC Branch2/LConn1

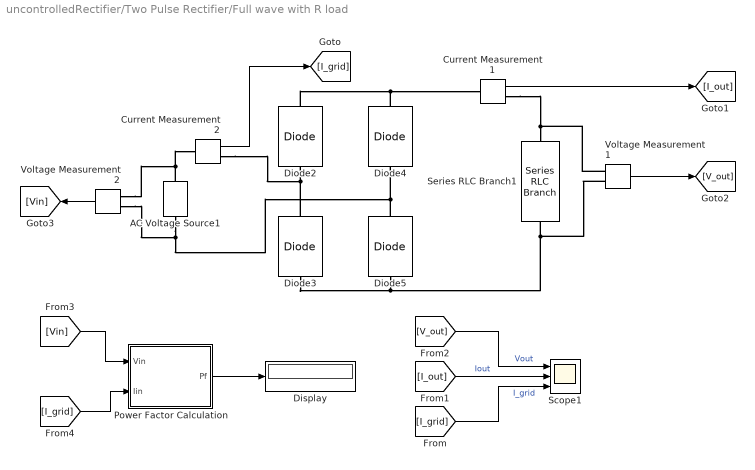
== system uncontrolledRectifier/Two Pulse Rectifier/Full wave with R load ==
  AC Voltage Source1 : spsACVoltageSourceLib/AC Voltage Source  Amplitude=220  Phase=0  Frequency=50  SampleTime=0  Measurements=None  BusType=swing  Pref=10e3  Qref=0  Qmin=-inf  Qmax=+inf
  Current Measurement1 : spsCurrentMeasurementLib/Current Measurement  PhasorSimulation=off  OutputType=Complex  PSBequivalent=0
  Current Measurement2 : spsCurrentMeasurementLib/Current Measurement  PhasorSimulation=off  OutputType=Complex  PSBequivalent=0
  Diode{2..5} (4 alike) : spsDiodeLib/Diode  Ron=0.001  Lon=0  Vf=0.8  IC=0  UseSnubber=0  Rs=500  Cs=250e-9  Measurements=off
  Display : Display
  Power Factor Calculation : Subsystem
  Scope1 : Scope  NumInputPorts=3
  Series RLC Branch1 : spsSeriesRLCBranchLib/Series RLC Branch  LConnTagsString=__new0  RConnTagsString=__new0  BranchType=R  Resistance=10  Inductance=1e-3  SetiL0=off  InitialCurrent=0  Capacitance=1e-6  Setx0=off  InitialVoltage=0  Measurements=None
  Voltage Measurement1 : spsVoltageMeasurementLib/Voltage Measurement  PhasorSimulation=off  OutputType=Complex  PSBequivalent=0
  Voltage Measurement2 : spsVoltageMeasurementLib/Voltage Measurement  PhasorSimulation=off  OutputType=Complex  PSBequivalent=0
  wires:
  Current Measurement1/1 -> [I_out]
  Voltage Measurement1/1 -> [V_out]
  Current Measurement2/1 -> [I_grid]
  [V_out] -> Scope1/1  "Vout"
  [I_out] -> Scope1/2  "Iout"
  [I_grid] -> Scope1/3  "I_grid"
  Voltage Measurement2/1 -> [Vin]
  [Vin] -> Power Factor Calculation/1(Vin)
  [I_grid] -> Power Factor Calculation/2(Iin)
  Power Factor Calculation/1(Pf) -> Display/1
  connections:
  Diode2/RConn1 -- Diode4/RConn1 -- Current Measurement1/LConn1
  Current Measurement1/RConn1 -- Voltage Measurement1/LConn1 -- Series RLC Branch1/LConn1
  Diode3/RConn1 -- Current Measurement2/RConn1 -- Diode2/LConn1
  Voltage Measurement1/LConn2 -- Diode3/LConn1 -- Diode5/LConn1 -- Series RLC Branch1/RConn1
  Diode5/RConn1 -- Voltage Measurement2/LConn2 -- AC Voltage Source1/LConn1 -- Diode4/LConn1
  AC Voltage Source1/RConn1 -- Voltage Measurement2/LConn1 -- Current Measurement2/LConn1

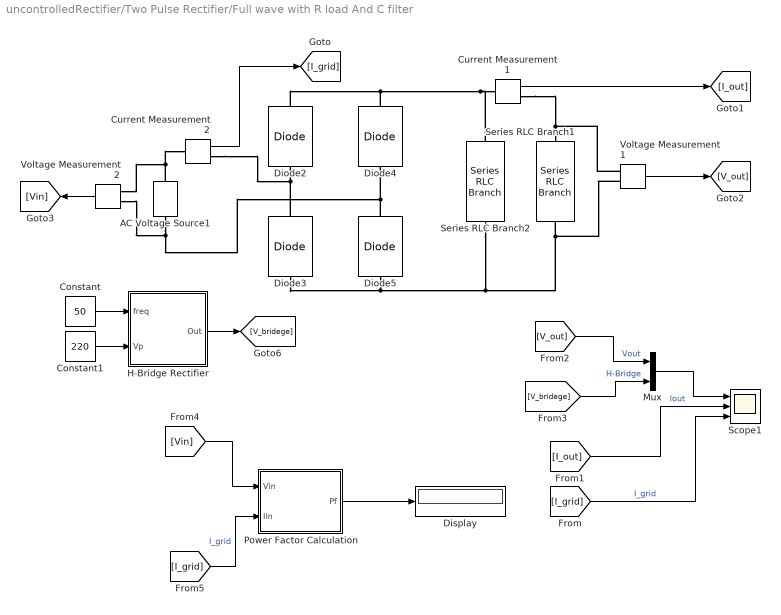
== system uncontrolledRectifier/Two Pulse Rectifier/Full wave with R load And C filter ==
  AC Voltage Source1 : spsACVoltageSourceLib/AC Voltage Source  Amplitude=220  Phase=0  Frequency=50  SampleTime=0  Measurements=None  BusType=swing  Pref=10e3  Qref=0  Qmin=-inf  Qmax=+inf
  Constant : Constant  Value=50
  Constant1 : Constant  Value=220
  Current Measurement1 : spsCurrentMeasurementLib/Current Measurement  PhasorSimulation=off  OutputType=Complex  PSBequivalent=0
  Current Measurement2 : spsCurrentMeasurementLib/Current Measurement  PhasorSimulation=off  OutputType=Complex  PSBequivalent=0
  Diode{2..5} (4 alike) : spsDiodeLib/Diode  Ron=0.001  Lon=0  Vf=0.8  IC=0  UseSnubber=0  Rs=500  Cs=250e-9  Measurements=off
  Display : Display
  H-Bridge Rectifier : Subsystem
  Mux : Mux  Inputs=2
  Power Factor Calculation : Subsystem
  Scope1 : Scope  NumInputPorts=3
  Series RLC Branch1 : spsSeriesRLCBranchLib/Series RLC Branch  LConnTagsString=__new0  RConnTagsString=__new0  BranchType=R  Resistance=10  Inductance=1e-3  SetiL0=off  InitialCurrent=0  Capacitance=1e-6  Setx0=off  InitialVoltage=0  Measurements=None
  Series RLC Branch2 : spsSeriesRLCBranchLib/Series RLC Branch  LConnTagsString=__new0  RConnTagsString=__new0  BranchType=C  Resistance=10  Inductance=1e-3  SetiL0=off  InitialCurrent=0  Capacitance=8e-3  Setx0=off  InitialVoltage=0  Measurements=None
  Voltage Measurement1 : spsVoltageMeasurementLib/Voltage Measurement  PhasorSimulation=off  OutputType=Complex  PSBequivalent=0
  Voltage Measurement2 : spsVoltageMeasurementLib/Voltage Measurement  PhasorSimulation=off  OutputType=Complex  PSBequivalent=0
  wires:
  [I_grid] -> Scope1/3  "I_grid"
  [I_out] -> Scope1/2  "Iout"
  [V_out] -> Mux/1  "Vout"
  Current Measurement2/1 -> [I_grid]
  Voltage Measurement1/1 -> [V_out]
  Current Measurement1/1 -> [I_out]
  [V_bridege] -> Mux/2  "H-Bridge"
  Mux/1 -> Scope1/1
  Constant/1 -> H-Bridge Rectifier/1(freq)
  H-Bridge Rectifier/1(Out) -> [V_bridege]
  Constant1/1 -> H-Bridge Rectifier/2(Vp)
  Voltage Measurement2/1 -> [Vin]
  [Vin] -> Power Factor Calculation/1(Vin)
  [I_grid] -> Power Factor Calculation/2(Iin)  "I_grid"
  Power Factor Calculation/1(Pf) -> Display/1
  connections:
  AC Voltage Source1/RConn1 -- Voltage Measurement2/LConn1 -- Current Measurement2/LConn1
  Diode4/LConn1 -- Voltage Measurement2/LConn2 -- AC Voltage Source1/LConn1 -- Diode5/RConn1
  Series RLC Branch1/RConn1 -- Diode5/LConn1 -- Diode3/LConn1 -- Series RLC Branch2/RConn1 -- Voltage Measurement1/LConn2
  Diode2/LConn1 -- Current Measurement2/RConn1 -- Diode3/RConn1
  Series RLC Branch1/LConn1 -- Voltage Measurement1/LConn1 -- Current Measurement1/RConn1
  Diode4/RConn1 -- Diode2/RConn1 -- Series RLC Branch2/LConn1 -- Current Measurement1/LConn1

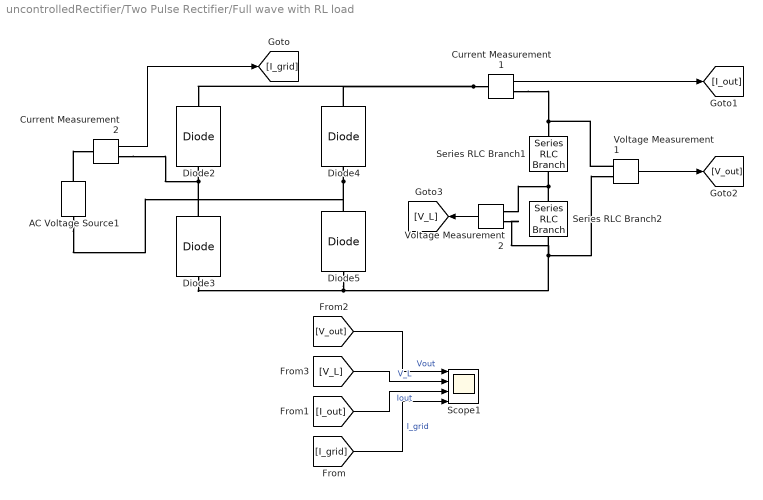
== system uncontrolledRectifier/Two Pulse Rectifier/Full wave with RL load ==
  AC Voltage Source1 : spsACVoltageSourceLib/AC Voltage Source  Amplitude=220  Phase=0  Frequency=50  SampleTime=0  Measurements=None  BusType=swing  Pref=10e3  Qref=0  Qmin=-inf  Qmax=+inf
  Current Measurement1 : spsCurrentMeasurementLib/Current Measurement  PhasorSimulation=off  OutputType=Complex  PSBequivalent=0
  Current Measurement2 : spsCurrentMeasurementLib/Current Measurement  PhasorSimulation=off  OutputType=Complex  PSBequivalent=0
  Diode{2..5} (4 alike) : spsDiodeLib/Diode  Ron=0.001  Lon=0  Vf=0.8  IC=0  UseSnubber=0  Rs=500  Cs=250e-9  Measurements=off
  Scope1 : Scope  NumInputPorts=4
  Series RLC Branch1 : spsSeriesRLCBranchLib/Series RLC Branch  LConnTagsString=__new0  RConnTagsString=__new0  BranchType=R  Resistance=10  Inductance=1e-3  SetiL0=off  InitialCurrent=0  Capacitance=1e-6  Setx0=off  InitialVoltage=0  Measurements=None
  Series RLC Branch2 : spsSeriesRLCBranchLib/Series RLC Branch  LConnTagsString=__new0  RConnTagsString=__new0  BranchType=L  Resistance=10  Inductance=100e-3  SetiL0=off  InitialCurrent=0  Capacitance=1e-6  Setx0=off  InitialVoltage=0  Measurements=None
  Voltage Measurement1 : spsVoltageMeasurementLib/Voltage Measurement  PhasorSimulation=off  OutputType=Complex  PSBequivalent=0
  Voltage Measurement2 : spsVoltageMeasurementLib/Voltage Measurement  PhasorSimulation=off  OutputType=Complex  PSBequivalent=0
  wires:
  [I_grid] -> Scope1/4  "I_grid"
  Voltage Measurement1/1 -> [V_out]
  [V_out] -> Scope1/1  "Vout"
  Current Measurement2/1 -> [I_grid]
  Current Measurement1/1 -> [I_out]
  [I_out] -> Scope1/3  "Iout"
  Voltage Measurement2/1 -> [V_L]
  [V_L] -> Scope1/2  "V_L"
  connections:
  Current Measurement1/LConn1 -- Diode2/RConn1 -- Diode4/RConn1
  Diode4/LConn1 -- AC Voltage Source1/LConn1 -- Diode5/RConn1
  Series RLC Branch1/LConn1 -- Current Measurement1/RConn1 -- Voltage Measurement1/LConn1
  Diode5/LConn1 -- Voltage Measurement2/LConn2 -- Series RLC Branch2/RConn1 -- Voltage Measurement1/LConn2 -- Diode3/LConn1
  Diode2/LConn1 -- Current Measurement2/RConn1 -- Diode3/RConn1
  AC Voltage Source1/RConn1 -- Current Measurement2/LConn1
  Series RLC Branch2/LConn1 -- Voltage Measurement2/LConn1 -- Series RLC Branch1/RConn1

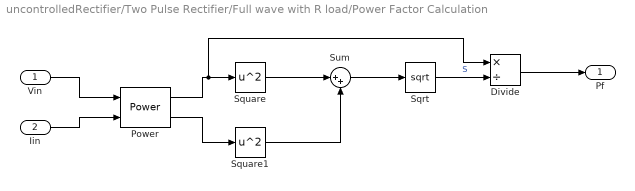
== system uncontrolledRectifier/Two Pulse Rectifier/Full wave with R load/Power Factor Calculation ==
  Vin : Inport
  Iin : Inport  Port=2
  Divide : Product  Inputs=*/
  Power : spsPowerLib/Power  Freq=60  Vinit=[1, 0]  Iinit=[1, 0]  Ts=0
      settings: SourceProductBaseCode=PS
  Sqrt : Sqrt  SaturateOnIntegerOverflow=on
  Square : Math  Operator=square  SaturateOnIntegerOverflow=on
  Square1 : Math  Operator=square  SaturateOnIntegerOverflow=on
  Sum : Sum  Inputs=|++
  Pf : Outport
  wires:
  Sum/1 -> Sqrt/1
  Power/1 -> Divide/1, Square/1
  Square/1 -> Sum/1
  Vin/1 -> Power/1
  Power/2 -> Square1/1
  Divide/1 -> Pf/1
  Square1/1 -> Sum/2
  Sqrt/1 -> Divide/2  "S"
  Iin/1 -> Power/2

== system uncontrolledRectifier/Two Pulse Rectifier/Full wave with R load And C filter/H-Bridge Rectifier ==
  freq : Inport
  Vp : Inport  Port=2
  2*pi : Gain  Gain=2*pi
  Abs : Abs
  Clock : Clock
  Product : Product
  Product1 : Product
  Sin : Trigonometry
  Out : Outport
  wires:
  Product1/1 -> Abs/1
  Product/1 -> Sin/1
  Clock/1 -> Product/1
  freq/1 -> 2*pi/1
  2*pi/1 -> Product/2
  Abs/1 -> Out/1
  Sin/1 -> Product1/1
  Vp/1 -> Product1/2

== system uncontrolledRectifier/Two Pulse Rectifier/Full wave with R load And C filter/Power Factor Calculation ==
  Vin : Inport
  Iin : Inport  Port=2
  Divide : Product  Inputs=*/
  Power : spsPowerLib/Power  Freq=60  Vinit=[1, 0]  Iinit=[1, 0]  Ts=0
      settings: SourceProductBaseCode=PS
  Sqrt : Sqrt  SaturateOnIntegerOverflow=on
  Square : Math  Operator=square  SaturateOnIntegerOverflow=on
  Square1 : Math  Operator=square  SaturateOnIntegerOverflow=on
  Sum : Sum  Inputs=|++
  Pf : Outport
  wires:
  Sum/1 -> Sqrt/1
  Power/1 -> Divide/1, Square/1
  Square/1 -> Sum/1
  Vin/1 -> Power/1
  Power/2 -> Square1/1
  Divide/1 -> Pf/1
  Square1/1 -> Sum/2
  Sqrt/1 -> Divide/2  "S"
  Iin/1 -> Power/2
